simulink model "FuelCellWorkBench"  (Simulink 4.00)
settings: Solver=ode1  StartTime=0.0  StopTime=max(pwr_profile(:,1))  FixedStep=1  RelTol=1e-3
undefined symbols (not defined in the file or in its folder): cyc_elevation_init
libraries: lib_fuel_cell x1
settings Model: LastModifiedBy=tmarkel

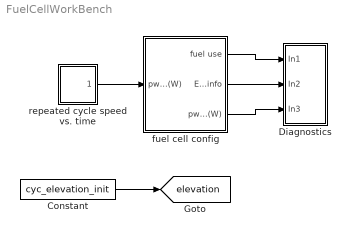
== system FuelCellWorkBench ==
  Constant : Constant  Value=cyc_elevation_init
  Diagnostics : Subsystem
      settings: RTWFcnNameOpts=Auto  RTWFileNameOpts=Auto
  fuel cell config : Subsystem  BlockChoice=fuel converter <fc> VT model
      settings: AttributesFormatString=%<BlockChoice>  TemplateBlock=lib_fuel_cell/fuel cell config  MemberBlocks="fuel converter <fc>  KTH fc model,fuel converter <fc> GCTool linkage,fuel converter <fc> VT model,fuel converter <fc> net model,fuel converter <fc> polarization curve model"  RTWFcnNameOpts=Auto  RTWFileNameOpts=Auto
  repeated cycle speed vs. time : Subsystem  mask(Repeating table){@1=pwr_profile(:,1), @2=pwr_profile(:,2)}
      mask prompts: @1 "Time values:"; @2 "Output values:"
      mask help:
      | Repeating table.
      | Enter values of time and output for first cycle.
      mask init:
      | period = max(@1); t = @1; y = @2;
      settings: RTWFcnNameOpts=Auto  RTWFileNameOpts=Auto
      mask Help: Repeats cycle given in table. Time values should be monotonically increasing.
  tag scope: elevation=global
  wires:
  repeated cycle speed vs. time/1(out_1) -> fuel cell config/1(pwr req'd at fc  output (W))
  fuel cell config/1(fuel use) -> Diagnostics/1(In1)
  fuel cell config/2(EO emis info) -> Diagnostics/2(In2)
  fuel cell config/3(pwr avail. to driveline (W)) -> Diagnostics/3(In3)
  Constant/1 -> [elevation]

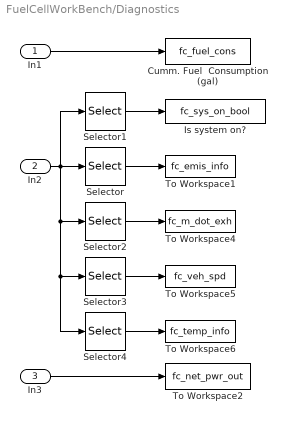
== system FuelCellWorkBench/Diagnostics ==
  In1 : Inport  Port=1  LatchInput=off
  In2 : Inport  Port=2  LatchInput=off
  In3 : Inport  Port=3  LatchInput=off
  Cumm. Fuel  Consumption (gal) : ToWorkspace  VariableName=fc_fuel_cons  SampleTime=-1  SaveFormat=Array
  Is system on? : ToWorkspace  VariableName=fc_sys_on_bool  SampleTime=-1  SaveFormat=Array
  Selector : Selector  InputType=Vector  ElementSrc=Internal  Elements=[2 3 4 5 8]  RowSrc=Internal  Rows=1  ColumnSrc=Internal  Columns=1  InputPortWidth=13
  Selector1 : Selector  InputType=Vector  ElementSrc=Internal  Elements=[1]  RowSrc=Internal  Rows=1  ColumnSrc=Internal  Columns=1  InputPortWidth=13
  Selector2 : Selector  InputType=Vector  ElementSrc=Internal  Elements=[6]  RowSrc=Internal  Rows=1  ColumnSrc=Internal  Columns=1  InputPortWidth=13
  Selector3 : Selector  InputType=Vector  ElementSrc=Internal  Elements=[8]  RowSrc=Internal  Rows=1  ColumnSrc=Internal  Columns=1  InputPortWidth=13
  Selector4 : Selector  InputType=Vector  ElementSrc=Internal  Elements=[10 11 12 13 7]  RowSrc=Internal  Rows=1  ColumnSrc=Internal  Columns=1  InputPortWidth=13
  To Workspace1 : ToWorkspace  VariableName=fc_emis_info  SampleTime=-1  SaveFormat=Array
  To Workspace2 : ToWorkspace  VariableName=fc_net_pwr_out  SampleTime=-1  SaveFormat=Array
  To Workspace4 : ToWorkspace  VariableName=fc_m_dot_exh  SampleTime=-1  SaveFormat=Array
  To Workspace5 : ToWorkspace  VariableName=fc_veh_spd  SampleTime=-1  SaveFormat=Array
  To Workspace6 : ToWorkspace  VariableName=fc_temp_info  SampleTime=-1  SaveFormat=Array
  wires:
  Selector4/1 -> To Workspace6/1
  Selector3/1 -> To Workspace5/1
  Selector2/1 -> To Workspace4/1
  Selector1/1 -> Is system on?/1
  Selector/1 -> To Workspace1/1
  In2/1 -> Selector4/1, Selector3/1, Selector2/1, Selector1/1, Selector/1
  In3/1 -> To Workspace2/1
  In1/1 -> Cumm. Fuel  Consumption (gal)/1

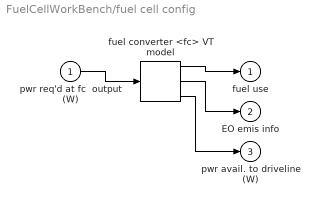
== system FuelCellWorkBench/fuel cell config ==
  pwr req'd at fc  output (W) : Inport  Port=1  LatchInput=off
  fuel converter <fc> VT model : lib_fuel_cell/fuel converter <fc> VT model
  fuel use : Outport  Port=1
  EO emis info : Outport  Port=2
  pwr avail. to driveline (W) : Outport  Port=3
  wires:
  pwr req'd at fc  output (W)/1 -> fuel converter <fc> VT model/1
  fuel converter <fc> VT model/1 -> fuel use/1
  fuel converter <fc> VT model/2 -> EO emis info/1
  fuel converter <fc> VT model/3 -> pwr avail. to driveline (W)/1

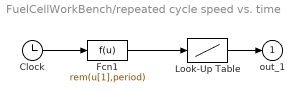
== system FuelCellWorkBench/repeated cycle speed vs. time ==
  Clock : Clock
      settings: DisplayTime=off  Decimation=10
  Fcn1 : Fcn  Expr=rem(u[1],period)
  Look-Up Table : Lookup  InputValues=t  OutputValues=y
  out_1 : Outport  Port=1  InitialOutput=0
  wires:
  Fcn1/1 -> Look-Up Table/1
  Clock/1 -> Fcn1/1
  Look-Up Table/1 -> out_1/1
